simulink model "SimulinkIoTThingSpeak_complete"  (R2026a)
settings: Solver=FixedStepAuto  StopTime=inf
undefined symbols (not defined in the file): Fi, SensorKnob, ThresholdKnob, Wi
libraries: arduinolib x5, arduinowifilib x2
settings Model: SimulationMode=external  SILPILModeSetting=veronly  ExtModeTrigDuration=2  TunableVars=SensorKnob,ThresholdKnob  TunableVarsStorageClass=ExportedGlobal,ExportedGlobal  TunableVarsTypeQualifier=const,const  Creator=AdePratamaSuryoKusum  LastModifiedBy=AdePratamaSuryoKusum
settings OptimizationCC: OptimizeBlockIOStorage=off  BufferReuse=off  GlobalBufferReuse=off  ExpressionFolding=off  EnableMemcpy=off  LocalBlockOutputs=off  OptimizeDataStoreBuffers=off  BusAssignmentInplaceUpdate=off  OptimizationLevel=level0
settings HardwareCC: ProdLargestAtomicInteger=Long  ProdLargestAtomicFloat=Double  ProdHWDeviceType=ARM Compatible->ARM Cortex
settings RTWCC: SystemTargetFile=ert.tlc  HardwareBoard=ESP32-WROOM (Arduino Compatible)  TLCOptions="-aInlineSetEventsForThisBaseRateFcn=TLC_FALSE -aSuppressMultiTaskScheduler=TLC_FALSE  -aRateBasedStepFcn=0"  Toolchain=ESP32  BuildConfiguration=Debug  Description=Embedded Coder
settings ERTTargetCC: ExtMode=on  ExtModeTransport=3.0  ExtModeAutomaticAllocSize=off  ExtModeStaticAllocSize=131072.0  ExtModeMexArgs=8  SupportContinuousTime=on  SupportVariableSizeSignals=on

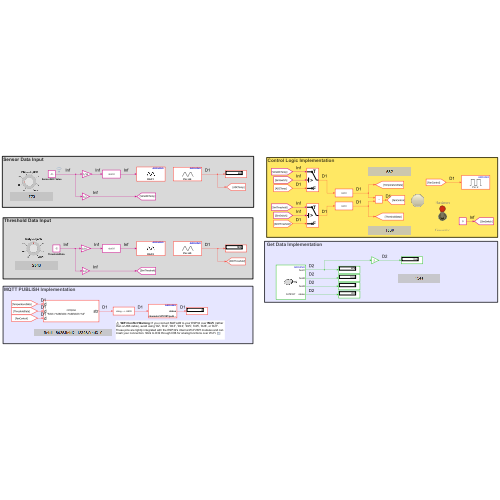
[thumbnail: Simulink's stored preview of the top-level diagram]
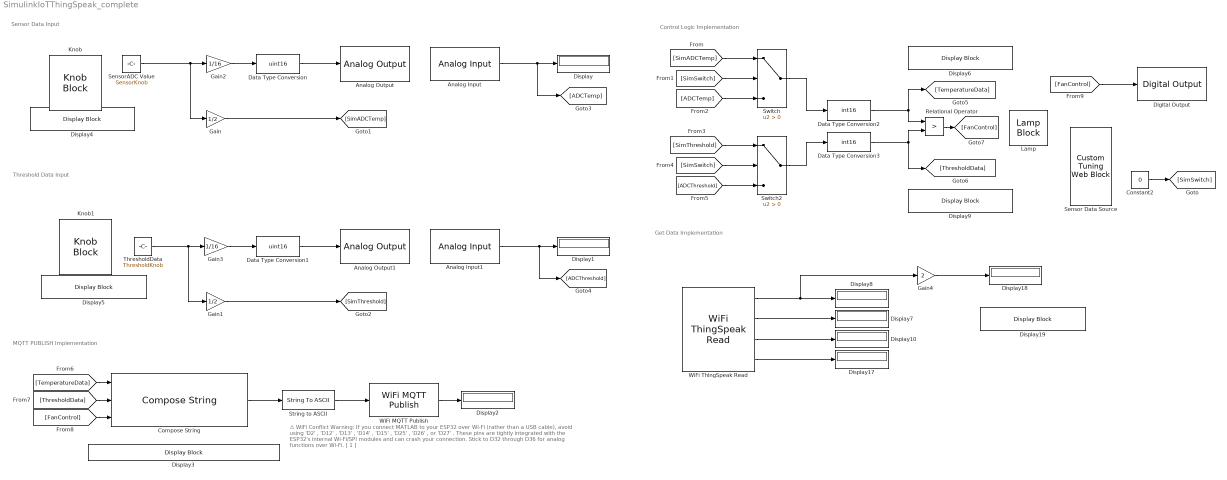
== system SimulinkIoTThingSpeak_complete ==
  note: Control Logic Implementation
  note: Threshold Data Input
  note: Get Data Implementation
  note: MQTT PUBLISH Implementation
  note: ⚠️ WiFi Conflict Warning: If you connect MATLAB to your ESP32 over Wi-Fi (rather than a USB cable), avoid using 'D2' , 'D12' , 'D13' , 'D14' , 'D15' , 'D25' , 'D26' , or 'D27' . These pins are tightly integrated with the ESP32's internal Wi-Fi/SPI modules and can crash your connection. Stick to D32 through D36 for analog functions over Wi-Fi. [ 1 ]
  note: Sensor Data Input
  Analog Input : arduinolib/Analog Input  pinNumber=4  ReadResultsOnly=off  ConversionTriggerSource=Software  ExternalTriggerType=uint32( 0 )  OutputDataType=uint16  EnableConversionCompleteNotify=off  EnableOuputStatus=off  SampleTime=0.01  blockPlatform=arduino
  Analog Input1 : arduinolib/Analog Input  pinNumber=5  ReadResultsOnly=off  ConversionTriggerSource=Software  ExternalTriggerType=uint32( 0 )  OutputDataType=uint16  EnableConversionCompleteNotify=off  EnableOuputStatus=off  SampleTime=0.01  blockPlatform=arduino
  Analog Output : arduinolib/Analog Output  blockPlatform=ARDUINO  DACpin=DAC1
  Analog Output1 : arduinolib/Analog Output  blockPlatform=ARDUINO  DACpin=DAC2
  Compose String : ComposeString  Format="\"field1=%d&field2=%d&field3=%d\""
  Constant2 : Constant  Value=0
  Data Type Conversion : DataTypeConversion  OutDataTypeStr=uint16  SaturateOnIntegerOverflow=off  RndMeth=Floor
  Data Type Conversion1 : DataTypeConversion  OutDataTypeStr=uint16  SaturateOnIntegerOverflow=off  RndMeth=Floor
  Data Type Conversion2 : DataTypeConversion  OutDataTypeStr=int16  SaturateOnIntegerOverflow=off  RndMeth=Floor
  Data Type Conversion3 : DataTypeConversion  OutDataTypeStr=int16  SaturateOnIntegerOverflow=off  RndMeth=Floor
  Digital Output : arduinolib/Digital Output  pinNumber=2  Direction=output  blockPlatform=arduino
  Display{,1..2,7..8,10,17..18} (8 alike) : Display
  Display{3,6,9,19} (4 alike) : DisplayBlock  LabelPosition=Hide  Transparency=1  GridColor=[0.502, 0.502, 0.502]
  Display4 : DisplayBlock  LabelPosition=Hide  Format=Integer  Transparency=1  GridColor=[0.502, 0.502, 0.502]
  Display5 : DisplayBlock  LabelPosition=Hide  Format=Integer  Transparency=1  GridColor=[0.502, 0.502, 0.502]
  Gain : Gain  Gain=1/2  OutDataTypeStr=int32
  Gain1 : Gain  Gain=1/2  OutDataTypeStr=int32
  Gain2 : Gain  Gain=1/16
  Gain3 : Gain  Gain=1/16
  Gain4 : Gain  Gain=2
  Knob : KnobBlock  ScaleMax=4095
  Knob1 : KnobBlock  ScaleMax=4095
  Lamp : LampBlock  LabelPosition=Hide  DefaultColor=[192.0, 192.0, 192.0]
  Relational Operator : RelationalOperator  Operator=>  OutDataTypeStr=boolean  RndMeth=Simplest  InputSameDT=off
  Sensor Data Source : CustomTuningWebBlock  LabelPosition=Hide  ShowInitialText=on  Configuration="{\"components\":[{\"name\":\"CustomSwitchStateComponent\",\"settings\":{\"position\":[0,0,1,1],\"showAllLabels\":1,\"states\":[{\"HitRegion\":{\"position\":[0,0,1,0.5]},\"Image\":{\"position\":[0,0.24928571428571428,0.5014285714285714,1],\"size\":[0.5014285714285714,1],\"src\":\"data:image\\/svg+xml;base64,PHN2ZyB4bWxucz0iaHR0cDovL3d3dy53My5vcmcvMjAwMC9zdmciIHhtbG5zOnhsaW5rPSJodHRwOi8vd3d3LnczLm9yZy8xOTk5L3hsaW5rIiB2aWV3Qm94PSIwIDAgMzguMDQgMTUwIj48ZGVmcz48c3R5bGU+LmNscy0xe2ZpbGw6dXJsKCNyYWRpYWwtZ3JhZGllbnQpO30uY2xzLTJ7ZmlsbDp1cmwoI3JhZGlhbC1ncmFkaWVudC0yKTt9LmNscy0ze2ZpbGw6dXJsKCNXaGl0ZV9CbGFjayk7fS5jbHMtNHtmaWxsOnVybCgjcmFkaWFsLWdyYWRpZW50LTMpO30uY2xzLTV7ZmlsbDojNWI1YjViO30uY2xzLTZ7ZmlsbDp1cmwoI3Jh ...(+3628 chars)\",\"srcOrientation\":\"Right\"},\"Label\":{\"color\":[0.5019607843137255,0.5019607843137255,0.5019607843137255],\"icon\":{\"size\":[0,0],\"src\":[],\"srcOrientation\":\"Right\"},\"iconOffset\":0,\"iconPlacement\":\"left\",\"opacity\":1,\"position\":[0.08,0.5],\"show\":true,\"text\":{\"content\":\"Hardware\",\"font\":\"Helvetica\"}},\"Value\":0},{\"HitRegion\":{\"position\":[0.5,0,1,0.5]},\"Image\":{\"position\":[0,0.24928571428571428,0.5014285714285714,1],\"size\":[0.5014285714285714,1],\"src\":\"data:image\\/svg+xml;base64,PHN2ZyB4bWxucz0iaHR0cDovL3d3dy53My5vcmcvMjAwMC9zdmciIHhtbG5zOnhsaW5rPSJodHRwOi8vd3d3LnczLm9yZy8xOTk5L3hsaW5rIiB2aWV3Qm94PSIwIDAgMzguMDQgMTUwIj48ZGVmcz48c3R5bGU+LmNscy0xe2ZpbGw6dXJsKCNyYWRpYWwtZ3JhZGllbnQpO30uY2xzLTJ7ZmlsbDp1cmwoI3JhZGlhbC1ncmFkaWVudC0yKTt9LmNscy0ze2ZpbGw6dXJsKCNXaGl0ZV9CbGFjayk7fS5jbHMtNHtmaWxsOnVybCgjcmFkaWFsLWdyYWRpZW50LTMpO30uY2xzLTV7ZmlsbDojNWI1YjViO30uY2xzLTZ7ZmlsbDp1cmwoI3Jh ...(+3556 chars)\",\"srcOrientation\":\"Right\"},\"Label\":{\"color\":[0.5019607843137255,0.5019607843137255,0.5019607843137255],\"icon\":{\"size\":[0,0],\"src\":[],\"srcOrientation\":\"Right\"},\"iconOffset\":0,\"iconPlacement\":\"left\",\"opacity\":1,\"position\":[0.92,0.5],\"show\":true,\"text\":{\"content\":\"Simulated\",\"font\":\"Helvetica\"}},\"Value\":1}]}},{\"name\":\"BackgroundImageComponent\",\"settings\":{\"image\":{\"size\":[70,135],\"src\":\"default\",\"srcOrientation\":\"Right\"},\"position\":[0,0,1,1],\"scaleMode\":\"0\"}},{\"name\":\"ForegroundImageComponent\",\"settings\":{\"image\":{\"size\":[0,0],\"src\":\"default\",\"srcOrientation\":[]},\"isForeground\":1,\"position\":[0,0,1,1],\"scaleMode\":\"0\"}}],\"derived\":{\"blockParameters\":{\"StatesJSON\":[{\"Label\":\"Hardware\",\"Value\":0},{\"Label\":\"Simulated\",\"Value\":1}],\"fixedAspectRatio\":\"on\"}},\"settings\":{\"BindingType\":\"param\",\"backgroundColor\":[0,0,0],\"backgroundOffset\":0.14,\"fixedAspectRatio\":\"on\",\"foregroundColor\":[0,0,0],\"showBackgroundColor\":false,\"variant\":\"toggle\",\"version\":\"R2024b\"},\"type\":\"Switch\"}"
  SensorADC Value : Constant  Value=SensorKnob  OutDataTypeStr=int32
  String to ASCII : StringToASCII  OutputVectorSize=128
  Switch : Switch  Criteria=u2 > Threshold  SaturateOnIntegerOverflow=off  InputSameDT=off
  Switch2 : Switch  Criteria=u2 > Threshold  SaturateOnIntegerOverflow=off  InputSameDT=off
  ThresholdData : Constant  Value=ThresholdKnob  OutDataTypeStr=int32
  WiFi MQTT Publish : arduinowifilib/WiFi MQTT Publish  BrokerService=ThingSpeak  TopicStr=channels/3478187/publish  RetainMsg=off  UpdateInterval=60  PrintDiagnosticMessages=off
  WiFi ThingSpeak Read : arduinowifilib/WiFi ThingSpeak Read  ChannelID_=3478187  Interfacetype_=Wi-Fi  ChannelAccess_=Private  ReadAPIKey_=YOUR_READ_API_KEY  FieldsToRead_=[1 2 3]  PrintDiagnosticMessages_=off  SampleTime_=15  blockPlatform=ARDUINO
  wires:
  SensorADC Value/1 -> Gain/1, Gain2/1
  ThresholdData/1 -> Gain3/1, Gain1/1
  Data Type Conversion/1 -> Analog Output/1
  Data Type Conversion1/1 -> Analog Output1/1
  Analog Input1/1 -> Display1/1, [ADCThreshold]
  Analog Input/1 -> [ADCTemp], Display/1
  String to ASCII/1 -> WiFi MQTT Publish/1
  Compose String/1 -> String to ASCII/1
  WiFi MQTT Publish/1 -> Display2/1
  Switch/1 -> Data Type Conversion2/1
  [SimSwitch] -> Switch/2
  [ADCTemp] -> Switch/3
  [SimADCTemp] -> Switch/1
  Constant2/1 -> [SimSwitch]
  Gain2/1 -> Data Type Conversion/1
  Gain3/1 -> Data Type Conversion1/1
  [ADCThreshold] -> Switch2/3
  [SimThreshold] -> Switch2/1
  [SimSwitch] -> Switch2/2
  Switch2/1 -> Data Type Conversion3/1
  Data Type Conversion2/1 -> [TemperatureData], Relational Operator/1
  Data Type Conversion3/1 -> Relational Operator/2, [ThresholdData]
  Relational Operator/1 -> [FanControl]
  [TemperatureData] -> Compose String/1
  [ThresholdData] -> Compose String/2
  [FanControl] -> Compose String/3
  Gain/1 -> [SimADCTemp]
  Gain1/1 -> [SimThreshold]
  [FanControl] -> Digital Output/1
  WiFi ThingSpeak Read/1 -> Gain4/1, Display8/1
  WiFi ThingSpeak Read/2 -> Display7/1
  WiFi ThingSpeak Read/3 -> Display10/1
  WiFi ThingSpeak Read/4 -> Display17/1
  Gain4/1 -> Display18/1
